simulink model "top_model"  (R2020b)
settings: Solver=VariableStepAuto  StartTime=0.0  StopTime=10.0  RelTol=1e-3  EnableMultiTasking=on
settings Model: Creator=The MathWorks, Inc.  LastModifiedBy=zhoutinglin
settings DataIOCC: LimitDataPoints=on  ReturnWorkspaceOutputs=off
settings OptimizationCC: LifeSpan=inf
settings DebuggingCC: AllowSymbolicDim=off  SFUnexpectedBacktrackingDiag=warning  SFNoUnconditionalDefaultTransitionDiag=warning  SFExecutionAtInitializationDiag=none  ArithmeticOperatorsInVariantConditions=warning
settings ModelReferenceCC: PropagateSignalLabelsOutOfModel=off
settings SFSimCC: SimUseLocalCustomCode=off  CustomCodeUndefinedFunction=UseInterfaceOnly
settings RTWCC: RTWUseLocalCustomCode=off
settings CodeAppCC: StateflowObjectComments=on
settings GRTTargetCC: TargetLangStandard=C89/C90 (ANSI)
settings ConfigComp: CovMetricSettings=dw  CovSaveCumulativeToWorkspaceVar=on  CovSaveSingleToWorkspaceVar=on  CovExternalEMLEnable=off

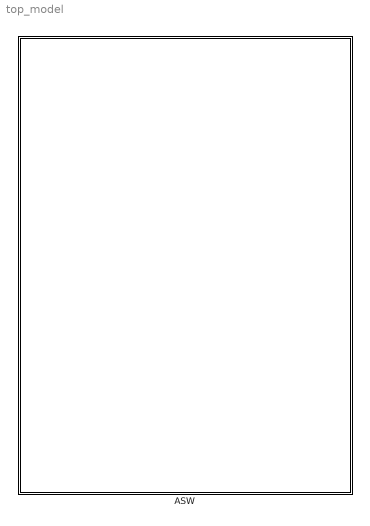
== system top_model ==
  ASW : Subsystem

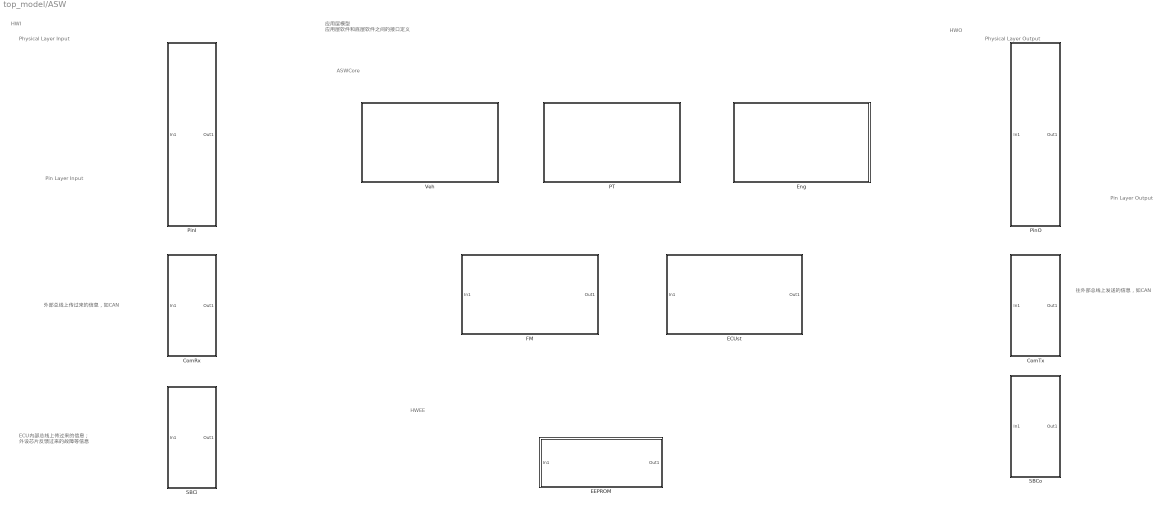
== system top_model/ASW ==
  note: Physical Layer Input
  note: HWO
  note: HWI
  note: Pin Layer Input
  note: ECU内部总线上传过来的信息；
      | 外设芯片反馈过来的故障等信息
  note: ASWCore
  note: Pin Layer Output
  note: 应用层模型
      | 应用层软件和底层软件之间的接口定义
  note: Physical Layer Output
  note: 外部总线上传过来的信息，如CAN
  note: 往外部总线上发送的信息，如CAN
  note: HWEE
  ComRx : Subsystem
  ComTx : Subsystem
  ECUst : Subsystem
  EEPROM : Subsystem
  Eng : Subsystem
  FM : Subsystem
  PT : Subsystem
  PinI : Subsystem
  PinO : Subsystem
  SBCi : Subsystem
  SBCo : Subsystem
  Veh : Subsystem

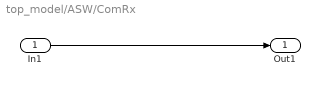
== system top_model/ASW/ComRx ==
  In1 : Inport
  Out1 : Outport  VectorParamsAs1DForOutWhenUnconnected=off
  wires:
  In1/1 -> Out1/1

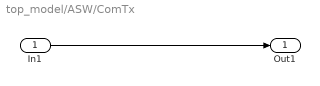
== system top_model/ASW/ComTx ==
  In1 : Inport
  Out1 : Outport  VectorParamsAs1DForOutWhenUnconnected=off
  wires:
  In1/1 -> Out1/1

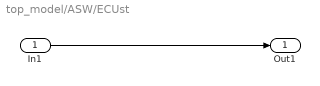
== system top_model/ASW/ECUst ==
  In1 : Inport
  Out1 : Outport  VectorParamsAs1DForOutWhenUnconnected=off
  wires:
  In1/1 -> Out1/1

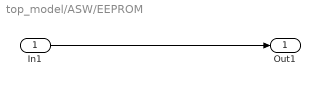
== system top_model/ASW/EEPROM ==
  In1 : Inport
  Out1 : Outport  VectorParamsAs1DForOutWhenUnconnected=off
  wires:
  In1/1 -> Out1/1

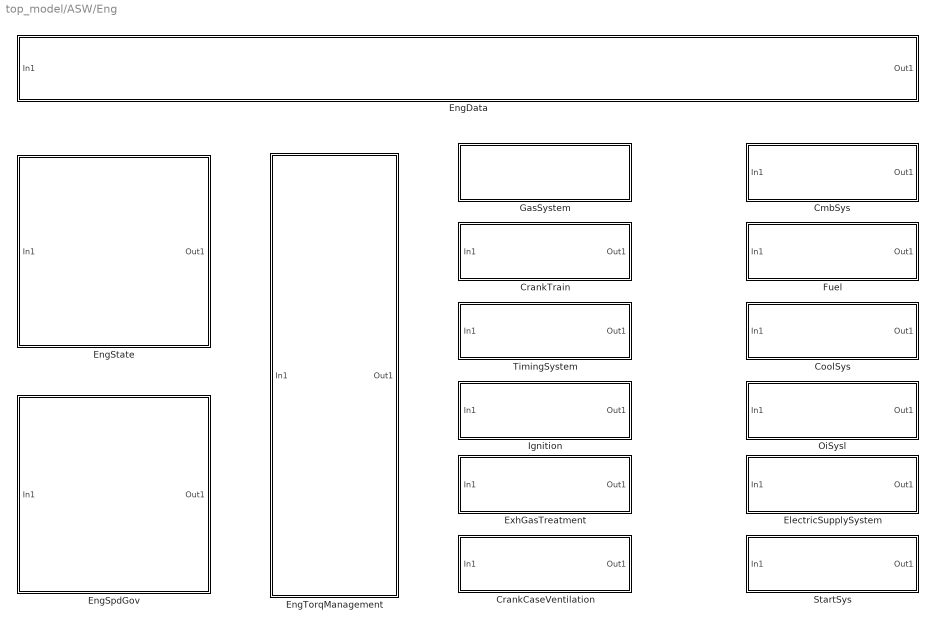
== system top_model/ASW/Eng ==
  CmbSys : Subsystem
  CoolSys : Subsystem
  CrankCaseVentilation : Subsystem
  CrankTrain : Subsystem
  ElectricSupplySystem : Subsystem
  EngData : Subsystem
  EngSpdGov : Subsystem
  EngState : Subsystem
  EngTorqManagement : Subsystem
  ExhGasTreatment : Subsystem
  Fuel : Subsystem
  GasSystem : Subsystem
  Ignition : Subsystem
  OiSysl : Subsystem
  StartSys : Subsystem
  TimingSystem : Subsystem

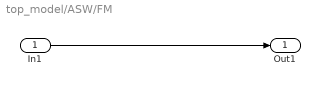
== system top_model/ASW/FM ==
  In1 : Inport
  Out1 : Outport  VectorParamsAs1DForOutWhenUnconnected=off
  wires:
  In1/1 -> Out1/1

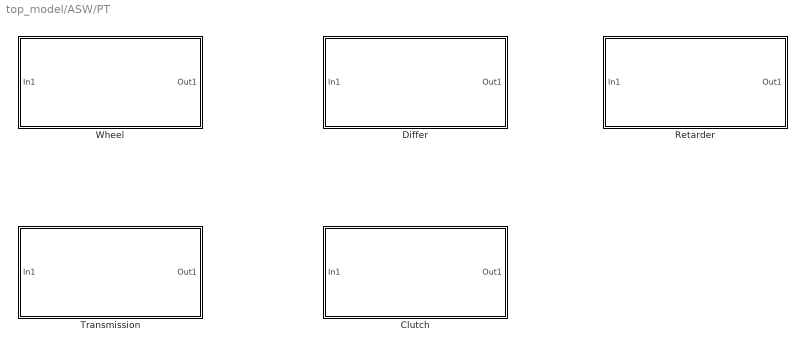
== system top_model/ASW/PT ==
  Clutch : Subsystem
  Differ : Subsystem
  Retarder : Subsystem
  Transmission : Subsystem
  Wheel : Subsystem

== system top_model/ASW/PinI ==
  In1 : Inport
  Out1 : Outport  VectorParamsAs1DForOutWhenUnconnected=off
  wires:
  In1/1 -> Out1/1

== system top_model/ASW/PinO ==
  In1 : Inport
  Out1 : Outport  VectorParamsAs1DForOutWhenUnconnected=off
  wires:
  In1/1 -> Out1/1

== system top_model/ASW/SBCi ==
  In1 : Inport
  Out1 : Outport  VectorParamsAs1DForOutWhenUnconnected=off
  wires:
  In1/1 -> Out1/1

== system top_model/ASW/SBCo ==
  In1 : Inport
  Out1 : Outport  VectorParamsAs1DForOutWhenUnconnected=off
  wires:
  In1/1 -> Out1/1

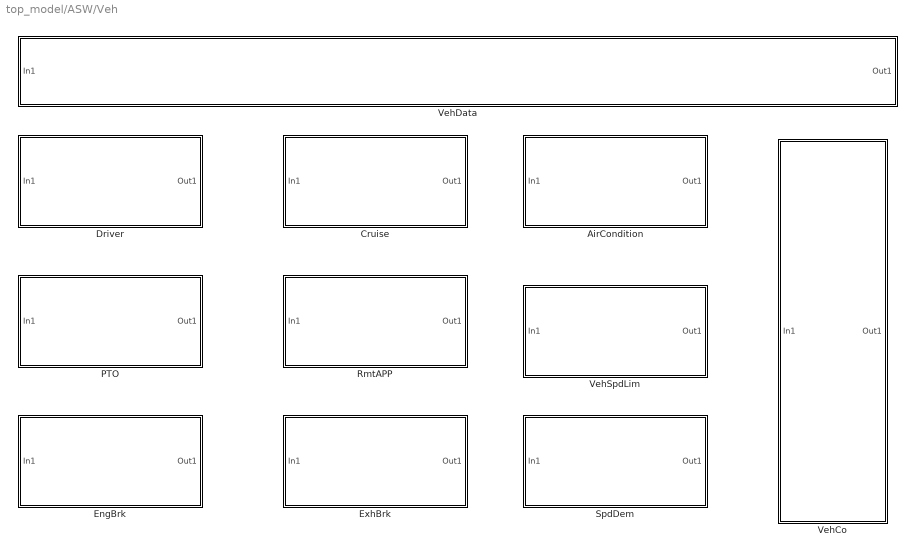
== system top_model/ASW/Veh ==
  AirCondition : Subsystem
  Cruise : Subsystem
  Driver : Subsystem
  EngBrk : Subsystem
  ExhBrk : Subsystem
  PTO : Subsystem
  RmtAPP : Subsystem
  SpdDem : Subsystem
  VehCo : Subsystem
  VehData : Subsystem
  VehSpdLim : Subsystem

== system top_model/ASW/Eng/CmbSys ==
  note: All of the demand comes from here: air pressure demand, injection quantity and injection time; smoke limit
  In1 : Inport
  Out1 : Outport  VectorParamsAs1DForOutWhenUnconnected=off
  wires:
  In1/1 -> Out1/1

== system top_model/ASW/Eng/CoolSys ==
  In1 : Inport
  Out1 : Outport  VectorParamsAs1DForOutWhenUnconnected=off
  wires:
  In1/1 -> Out1/1

== system top_model/ASW/Eng/CrankCaseVentilation ==
  In1 : Inport
  Out1 : Outport  VectorParamsAs1DForOutWhenUnconnected=off
  wires:
  In1/1 -> Out1/1

== system top_model/ASW/Eng/CrankTrain ==
  In1 : Inport
  Out1 : Outport  VectorParamsAs1DForOutWhenUnconnected=off
  wires:
  In1/1 -> Out1/1

== system top_model/ASW/Eng/ElectricSupplySystem ==
  In1 : Inport
  Out1 : Outport  VectorParamsAs1DForOutWhenUnconnected=off
  wires:
  In1/1 -> Out1/1

== system top_model/ASW/Eng/EngData ==
  In1 : Inport
  Out1 : Outport  VectorParamsAs1DForOutWhenUnconnected=off
  wires:
  In1/1 -> Out1/1

== system top_model/ASW/Eng/EngSpdGov ==
  In1 : Inport
  Out1 : Outport  VectorParamsAs1DForOutWhenUnconnected=off
  wires:
  In1/1 -> Out1/1

== system top_model/ASW/Eng/EngState ==
  In1 : Inport
  Out1 : Outport  VectorParamsAs1DForOutWhenUnconnected=off
  wires:
  In1/1 -> Out1/1

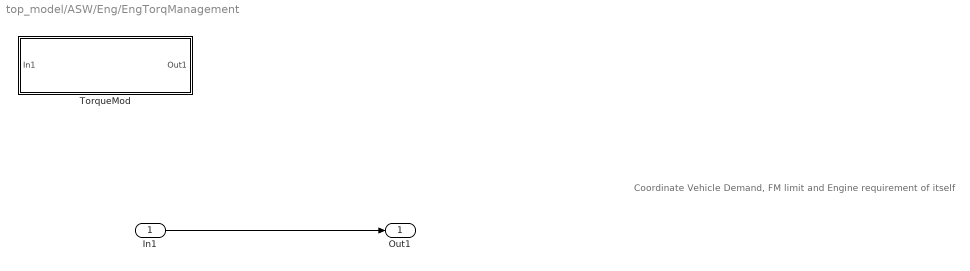
== system top_model/ASW/Eng/EngTorqManagement ==
  note: Coordinate Vehicle Demand, FM limit and Engine requirement of itself
  In1 : Inport
  TorqueMod : Subsystem
  Out1 : Outport  VectorParamsAs1DForOutWhenUnconnected=off
  wires:
  In1/1 -> Out1/1

== system top_model/ASW/Eng/ExhGasTreatment ==
  In1 : Inport
  Out1 : Outport  VectorParamsAs1DForOutWhenUnconnected=off
  wires:
  In1/1 -> Out1/1

== system top_model/ASW/Eng/Fuel ==
  In1 : Inport
  Out1 : Outport  VectorParamsAs1DForOutWhenUnconnected=off
  wires:
  In1/1 -> Out1/1

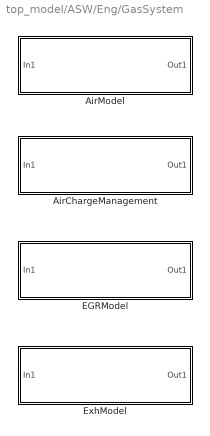
== system top_model/ASW/Eng/GasSystem ==
  AirChargeManagement : Subsystem
  AirModel : Subsystem
  EGRModel : Subsystem
  ExhModel : Subsystem

== system top_model/ASW/Eng/Ignition ==
  In1 : Inport
  Out1 : Outport  VectorParamsAs1DForOutWhenUnconnected=off
  wires:
  In1/1 -> Out1/1

== system top_model/ASW/Eng/OiSysl ==
  In1 : Inport
  Out1 : Outport  VectorParamsAs1DForOutWhenUnconnected=off
  wires:
  In1/1 -> Out1/1

== system top_model/ASW/Eng/StartSys ==
  In1 : Inport
  Out1 : Outport  VectorParamsAs1DForOutWhenUnconnected=off
  wires:
  In1/1 -> Out1/1

== system top_model/ASW/Eng/TimingSystem ==
  In1 : Inport
  Out1 : Outport  VectorParamsAs1DForOutWhenUnconnected=off
  wires:
  In1/1 -> Out1/1

== system top_model/ASW/PT/Clutch ==
  In1 : Inport
  Out1 : Outport  VectorParamsAs1DForOutWhenUnconnected=off
  wires:
  In1/1 -> Out1/1

== system top_model/ASW/PT/Differ ==
  In1 : Inport
  Out1 : Outport  VectorParamsAs1DForOutWhenUnconnected=off
  wires:
  In1/1 -> Out1/1

== system top_model/ASW/PT/Retarder ==
  In1 : Inport
  Out1 : Outport  VectorParamsAs1DForOutWhenUnconnected=off
  wires:
  In1/1 -> Out1/1

== system top_model/ASW/PT/Transmission ==
  In1 : Inport
  Out1 : Outport  VectorParamsAs1DForOutWhenUnconnected=off
  wires:
  In1/1 -> Out1/1

== system top_model/ASW/PT/Wheel ==
  In1 : Inport
  Out1 : Outport  VectorParamsAs1DForOutWhenUnconnected=off
  wires:
  In1/1 -> Out1/1

== system top_model/ASW/Veh/AirCondition ==
  In1 : Inport
  Out1 : Outport  VectorParamsAs1DForOutWhenUnconnected=off
  wires:
  In1/1 -> Out1/1

== system top_model/ASW/Veh/Cruise ==
  In1 : Inport
  Out1 : Outport  VectorParamsAs1DForOutWhenUnconnected=off
  wires:
  In1/1 -> Out1/1

== system top_model/ASW/Veh/Driver ==
  In1 : Inport
  Out1 : Outport  VectorParamsAs1DForOutWhenUnconnected=off
  wires:
  In1/1 -> Out1/1

== system top_model/ASW/Veh/EngBrk ==
  In1 : Inport
  Out1 : Outport  VectorParamsAs1DForOutWhenUnconnected=off
  wires:
  In1/1 -> Out1/1

== system top_model/ASW/Veh/ExhBrk ==
  In1 : Inport
  Out1 : Outport  VectorParamsAs1DForOutWhenUnconnected=off
  wires:
  In1/1 -> Out1/1

== system top_model/ASW/Veh/PTO ==
  In1 : Inport
  Out1 : Outport  VectorParamsAs1DForOutWhenUnconnected=off
  wires:
  In1/1 -> Out1/1

== system top_model/ASW/Veh/RmtAPP ==
  In1 : Inport
  Out1 : Outport  VectorParamsAs1DForOutWhenUnconnected=off
  wires:
  In1/1 -> Out1/1

== system top_model/ASW/Veh/SpdDem ==
  In1 : Inport
  Out1 : Outport  VectorParamsAs1DForOutWhenUnconnected=off
  wires:
  In1/1 -> Out1/1

== system top_model/ASW/Veh/VehCo ==
  note: Coordinate all of the Torque demand and Speed demand for Engine
  In1 : Inport
  Out1 : Outport  VectorParamsAs1DForOutWhenUnconnected=off
  wires:
  In1/1 -> Out1/1

== system top_model/ASW/Veh/VehData ==
  In1 : Inport
  Out1 : Outport  VectorParamsAs1DForOutWhenUnconnected=off
  wires:
  In1/1 -> Out1/1

== system top_model/ASW/Veh/VehSpdLim ==
  In1 : Inport
  Out1 : Outport  VectorParamsAs1DForOutWhenUnconnected=off
  wires:
  In1/1 -> Out1/1

== system top_model/ASW/Eng/EngTorqManagement/TorqueMod ==
  note: Torque Model: Main Quantity Calculation
  In1 : Inport
  Out1 : Outport  VectorParamsAs1DForOutWhenUnconnected=off
  wires:
  In1/1 -> Out1/1

== system top_model/ASW/Eng/GasSystem/AirChargeManagement ==
  In1 : Inport
  Out1 : Outport  VectorParamsAs1DForOutWhenUnconnected=off
  wires:
  In1/1 -> Out1/1

== system top_model/ASW/Eng/GasSystem/AirModel ==
  In1 : Inport
  Out1 : Outport  VectorParamsAs1DForOutWhenUnconnected=off
  wires:
  In1/1 -> Out1/1

== system top_model/ASW/Eng/GasSystem/EGRModel ==
  In1 : Inport
  Out1 : Outport  VectorParamsAs1DForOutWhenUnconnected=off
  wires:
  In1/1 -> Out1/1

== system top_model/ASW/Eng/GasSystem/ExhModel ==
  In1 : Inport
  Out1 : Outport  VectorParamsAs1DForOutWhenUnconnected=off
  wires:
  In1/1 -> Out1/1
